simulink subsystem "IdealVoltageSource"  (R2025b)
settings: Solver=VariableStepAuto  StartTime=0.0  StopTime=10.0  RelTol=1e-3
undefined symbols (not defined in the file): BattCurr, BattPwr, BattSoc, BattVolt, PlntBattIdealSoc, PlntBattIdealVolt, PlntBattNumCellSer
settings Model: ModifiedByFormat=The MathWorks, Inc.  Creator=The MathWorks, Inc.  LastModifiedBy=The MathWorks, Inc.
settings SolverCC: MaxZcPerStep=1.0
settings OptimizationCC: ReuseModelBlockBuffer=off
settings DebuggingCC: UnconnectedInputMsg=warning  UnconnectedOutputMsg=warning  UnconnectedLineMsg=warning
settings ModelReferenceCC: EnableRefExpFcnMdlSchedulingChecks=on
settings RTWCC: GPUComputeCapability=3.5  DLArmComputeVersion=19.05

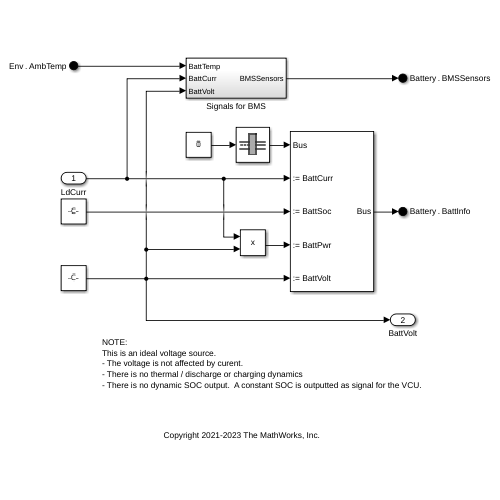
[thumbnail: Simulink's stored preview of the top-level diagram]
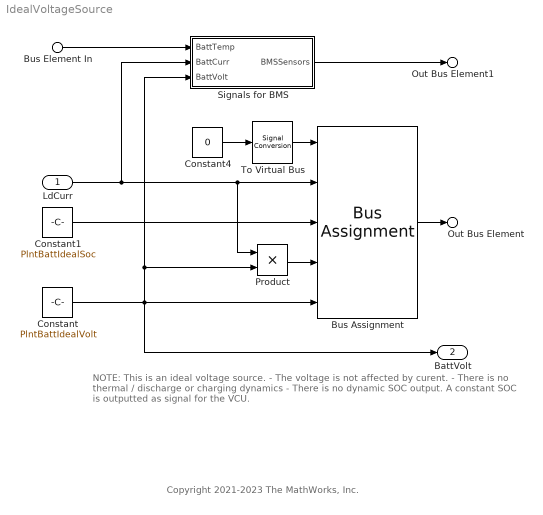
== system IdealVoltageSource ==
  note: NOTE:
      | This is an ideal voltage source.
      | - The voltage is not affected by curent.
      | - There is no thermal / discharge or charging dynamics
      | - There is no dynamic SOC output.  A constant SOC is outputted as signal for the VCU.
  note: Copyright 2021-2023 The MathWorks, Inc.
  LdCurr : Inport
  Bus Element In : Inport  Port=2  PortName=Env  Element=AmbTemp
  Bus Assignment : BusAssignment  AssignedSignals=BattCurr,BattSoc,BattPwr,BattVolt
  Constant : Constant  Value=PlntBattIdealVolt  SampleTime=-1
  Constant1 : Constant  Value=PlntBattIdealSoc  SampleTime=-1
  Constant4 : Constant  Value=0  OutDataTypeStr=Bus: BattInfoBUS  SampleTime=Inf
  Product : Product
  Signals for BMS : Subsystem
  To Virtual Bus : SignalConversion  ConversionOutput=Virtual bus  OverrideOpt=off
  Out Bus Element : Outport  PortName=Battery  Element=BattInfo
  Out Bus Element1 : Outport  PortName=Battery  Element=BMSSensors
  BattVolt : Outport  Port=2  VectorParamsAs1DForOutWhenUnconnected=off
  wires:
  Constant/1 -> Bus Assignment/5, BattVolt/1, Product/2, Signals for BMS/3(BattVolt)
  Bus Element In/1 -> Signals for BMS/1(BattTemp)
  LdCurr/1 -> Signals for BMS/2(BattCurr), Bus Assignment/2, Product/1
  Constant1/1 -> Bus Assignment/3
  Signals for BMS/1(BMSSensors) -> Out Bus Element1/1
  To Virtual Bus/1 -> Bus Assignment/1
  Constant4/1 -> To Virtual Bus/1
  Bus Assignment/1 -> Out Bus Element/1
  Product/1 -> Bus Assignment/4

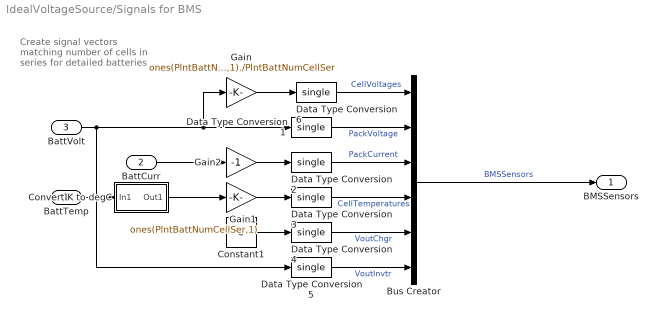
== system IdealVoltageSource/Signals for BMS ==
  note: Create signal vectors
      | matching number of
      | cells in series for
      | detailed batteries
  BattTemp : Inport
  BattCurr : Inport  Port=2
  BattVolt : Inport  Port=3
  Bus Creator : BusCreator  Inputs=6
  Constant1 : Constant  Value=0
  Convert K to degC : Subsystem
  Data Type Conversion{1..6} (6 alike) : DataTypeConversion  OutDataTypeStr=single  SaturateOnIntegerOverflow=off  RndMeth=Floor
  Gain : Gain  Gain=ones(PlntBattNumCellSer,1)./PlntBattNumCellSer
  Gain1 : Gain  Gain=ones(PlntBattNumCellSer,1)
  Gain2 : Gain  Gain=-1
  BMSSensors : Outport
  wires:
  BattCurr/1 -> Gain2/1
  Constant1/1 -> Data Type Conversion4/1
  BattVolt/1 -> Data Type Conversion1/1, Gain/1, Data Type Conversion5/1
  Gain/1 -> Data Type Conversion6/1
  BattTemp/1 -> Convert K to degC/1(In1)
  Data Type Conversion4/1 -> Bus Creator/5  "VoutChgr"
  Gain1/1 -> Data Type Conversion3/1
  Data Type Conversion5/1 -> Bus Creator/6  "VoutInvtr"
  Gain2/1 -> Data Type Conversion2/1
  Convert K to degC/1(Out1) -> Gain1/1
  Data Type Conversion1/1 -> Bus Creator/2  "PackVoltage"
  Data Type Conversion6/1 -> Bus Creator/1  "CellVoltages"
  Data Type Conversion2/1 -> Bus Creator/3  "PackCurrent"
  Data Type Conversion3/1 -> Bus Creator/4  "CellTemperatures"
  Bus Creator/1 -> BMSSensors/1  "BMSSensors"

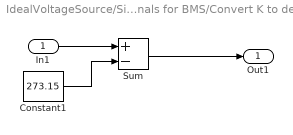
== system IdealVoltageSource/Signals for BMS/Convert K to degC ==
  In1 : Inport
  Constant1 : Constant  Value=273.15
  Sum : Sum  Inputs=+-
  Out1 : Outport
  wires:
  Sum/1 -> Out1/1
  Constant1/1 -> Sum/2
  In1/1 -> Sum/1
